simulink model "Soru3Gorev44"  (R2019a)
settings: Solver=VariableStepAuto  StartTime=0.0  StopTime=500  RelTol=1e-3
settings Model: Creator=handeyildirim  LastModifiedBy=handeyildirim

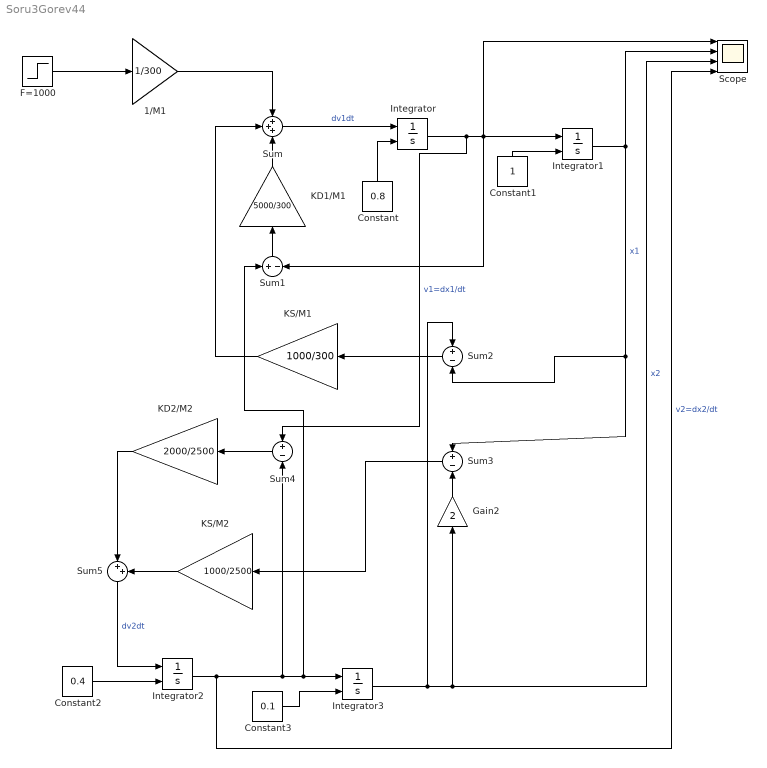
== system Soru3Gorev44 ==
  1/M1 : Gain  Gain=1/300
  Constant : Constant  Value=0.8
  Constant1 : Constant
  Constant2 : Constant  Value=0.4
  Constant3 : Constant  Value=0.1
  F=1000 : Step  Before=1000  After=1000  SampleTime=0
  Gain2 : Gain  Gain=2
  Integrator{,1..3} (4 alike) : Integrator  InitialConditionSource=external
  KD1/M1 : Gain  Gain=5000/300
  KD2/M2 : Gain  Gain=2000/2500
  KS/M1 : Gain  Gain=1000/300
  KS/M2 : Gain  Gain=1000/2500
  Scope : Scope  NumInputPorts=4
  Sum : Sum  Inputs=+++
  Sum{1..4} (4 alike) : Sum  Inputs=+-
  Sum5 : Sum  Inputs=|++
  wires:
  F=1000/1 -> 1/M1/1
  KD1/M1/1 -> Sum/3
  Constant/1 -> Integrator/2
  Sum/1 -> Integrator/1  "dv1dt"
  Sum1/1 -> KD1/M1/1
  Integrator/1 -> Sum4/1, Sum1/2, Scope/1, Integrator1/1  "v1=dx1/dt"
  Integrator1/1 -> Sum3/1, Sum2/2, Scope/2  "x1"
  1/M1/1 -> Sum/1
  Constant1/1 -> Integrator1/2
  KS/M1/1 -> Sum/2
  Sum2/1 -> KS/M1/1
  Gain2/1 -> Sum3/2
  Sum4/1 -> KD2/M2/1
  Sum3/1 -> KS/M2/1
  KS/M2/1 -> Sum5/2
  KD2/M2/1 -> Sum5/1
  Sum5/1 -> Integrator2/1  "dv2dt"
  Constant2/1 -> Integrator2/2
  Constant3/1 -> Integrator3/2
  Integrator2/1 -> Sum4/2, Sum1/1, Integrator3/1, Scope/4  "v2=dx2/dt"
  Integrator3/1 -> Scope/3, Gain2/1, Sum2/1  "x2"
